simulink model "punto4y5"  (R2024a)
settings: Solver=VariableStepAuto  StartTime=0.0  StopTime=50  RelTol=1e-3
libraries: fuzblock x3, slpidlib x1
settings Model: Creator=USER  LastModifiedBy=USER

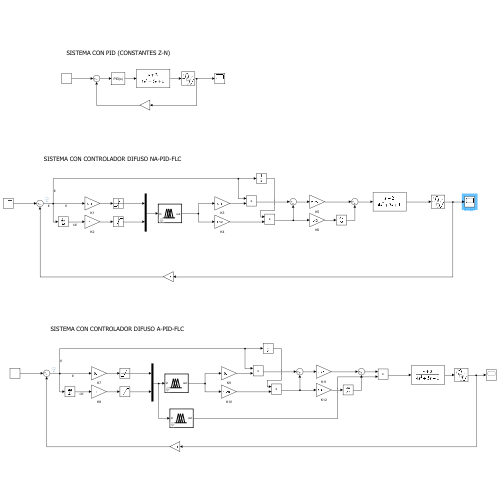
[thumbnail: Simulink's stored preview of the top-level diagram]
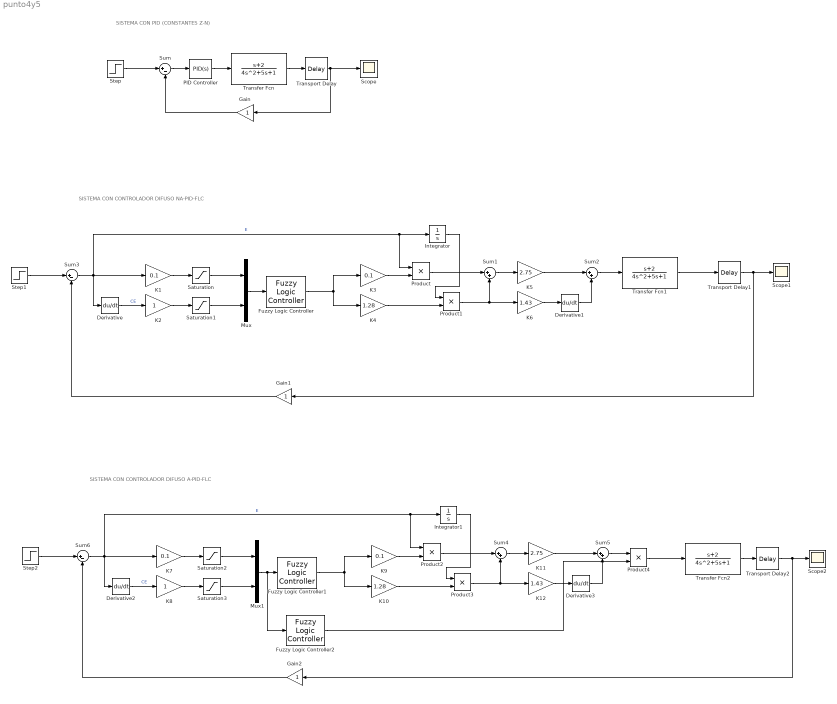
== system punto4y5 ==
  note: SISTEMA CON PID (CONSTANTES Z-N)
  note: SISTEMA CON CONTROLADOR DIFUSO NA-PID-FLC
  note: SISTEMA CON CONTROLADOR DIFUSO A-PID-FLC
  Derivative{,1..3} (4 alike) : Derivative
  Fuzzy Logic Controller : fuzblock/Fuzzy Logic  Controller  FIS='fuzzy_1.fis'  OutputSampleNumber=101  DataType=double  FuzzifiedInputs=off  RuleFiringStrengths=off  RuleOutputs=off  AggregatedOutputs=off  SimulateUsing=Interpreted execution  OutOfRangeInputValueMessage=warning  NoRuleFiredMessage=warning  EmptyOutputFuzzySetMessage=warning
  Fuzzy Logic Controller1 : fuzblock/Fuzzy Logic  Controller  FIS='fuzzy_1.fis'  OutputSampleNumber=101  DataType=double  FuzzifiedInputs=off  RuleFiringStrengths=off  RuleOutputs=off  AggregatedOutputs=off  SimulateUsing=Interpreted execution  OutOfRangeInputValueMessage=warning  NoRuleFiredMessage=warning  EmptyOutputFuzzySetMessage=warning
  Fuzzy Logic Controller2 : fuzblock/Fuzzy Logic  Controller  FIS='fuzzy_2.fis'  OutputSampleNumber=101  DataType=double  FuzzifiedInputs=off  RuleFiringStrengths=off  RuleOutputs=off  AggregatedOutputs=off  SimulateUsing=Interpreted execution  OutOfRangeInputValueMessage=warning  NoRuleFiredMessage=warning  EmptyOutputFuzzySetMessage=warning
  Gain : Gain
  Gain1 : Gain
  Gain2 : Gain
  Integrator : Integrator
  Integrator1 : Integrator
  K{1,3,7,9} (4 alike) : Gain  Gain=0.1
  K10 : Gain  Gain=1.28
  K11 : Gain  Gain=2.75
  K12 : Gain  Gain=1.43
  K2 : Gain
  K4 : Gain  Gain=1.28
  K5 : Gain  Gain=2.75
  K6 : Gain  Gain=1.43
  K8 : Gain
  Mux : Mux  Inputs=2
  Mux1 : Mux  Inputs=2
  PID Controller : slpidlib/PID Controller  Controller=PID  Form=Parallel  TimeDomain=Continuous-time  UseExternalTs=off  SampleTime=-1  IntegratorMethod=Forward Euler  FilterMethod=Forward Euler  ControllerParametersSource=internal  P=5.73  I=5  UseKiTs=off  D=1.43  UseExternalDerivativeSource=off  N=100  UseFilter=on  TunerSelectOption=Transfer Function Based (PID Tuner App)  InitialConditionSource=internal  InitialConditionForIntegrator=0  InitialConditionForFilter=0  DifferentiatorICPrevScaledInput=0  ExternalReset=none  TrackingMode=off  Kt=1  LimitOutput=off  SatLimitsSource=internal  UpperSaturationLimit=inf  LowerSaturationLimit=-inf  LinearizeAsGain=on  AntiWindupMode=none  Kb=1  LimitIntegrator=off  UpperIntegratorSaturationLimit=inf  LowerIntegratorSaturationLimit=-inf  POutMin=[]  POutMax=[]  IOutMin=[]  IOutMax=[]  DOutMin=[]  DOutMax=[]  NOutMin=[]  NOutMax=[]  SumOutMin=[]  SumOutMax=[]  SaturationOutMin=[]  SaturationOutMax=[]  PParamMin=[]  PParamMax=[]  IParamMin=[]  IParamMax=[]  DParamMin=[]  DParamMax=[]  NParamMin=[]  NParamMax=[]  KbParamMin=[]  KbParamMax=[]  KtParamMin=[]  KtParamMax=[]  KbOutMin=[]  KbOutMax=[]  KtOutMin=[]  KtOutMax=[]  IntegratorOutMin=[]  IntegratorOutMax=[]  FilterOutMin=[]  FilterOutMax=[]  SumI1OutMin=[]  SumI1OutMax=[]  SumI2OutMin=[]  SumI2OutMax=[]  SumI3OutMin=[]  SumI3OutMax=[]  SumI4OutMin=[]  SumI4OutMax=[]  SumDOutMin=[]  SumDOutMax=[]  DifferentiatorOutMin=[]  DifferentiatorOutMax=[]  FilterDiffOutCoefMin=[]  FilterDiffOutCoefMax=[]  ReciprocalOutMin=[]  ReciprocalOutMax=[]  SumDenOutMin=[]  SumDenOutMax=[]  SumNumOutMin=[]  SumNumOutMax=[]  DivideOutMin=[]  DivideOutMax=[]  UdiffTsProdOutMin=[]  UdiffTsProdOutMax=[]  NTsProdOutMin=[]  NTsProdOutMax=[]  UintegralTsProdOutMin=[]  UintegralTsProdOutMax=[]  UngainTsProdOutMin=[]  UngainTsProdOutMax=[]  ClampingZeroOutDataTypeStr=Inherit: Inherit via back propagation  ClampingZeroOutMin=[]  ClampingZeroOutMax=[]  FilterDenConstantOutDataTypeStr=Inherit: Inherit via back propagation  FilterDenConstantOutMin=[]  FilterDenConstantOutMax=[]  PCopyOutDataTypeStr=Inherit: Inherit via back propagation  PCopyOutMin=[]  PCopyOutMax=[]  NCopyOutDataTypeStr=Inherit: Inherit via back propagation  NCopyOutMin=[]  NCopyOutMax=[]  IntegratorContinuousStateAttributes=''  IntegratorStateMustResolveToSignalObject=off  IntegratorRTWStateStorageClass=Auto  FilterContinuousStateAttributes=''  FilterStateMustResolveToSignalObject=off  FilterRTWStateStorageClass=Auto  ParallelPVariant=InternalParameters  IdealPVariant=Disabled  IVariant=InternalParameters  DVariant=InternalParameters  IntegratorVariant=Continuous  SatVariant=Disabled  AWVariant=Passthrough  PCopyVariant=Disabled  TRVariant=Disabled  FdbkBlocksVariant=Forward  IdealPFdbkVariant=Disabled  SatFdbkVariant=Disabled  DerivativeFilterVariant=ContFilter  NVariant=InternalParameters  NCopyVariant=Disabled  FilterICVariant=InternalICsFilter  IntegratorICVariant=InternalICs  ExternalResetVariant=Disabled  TRSumVariant=Passthrough  SumFdbkVariant=Disabled  SumVariant=Sum_PID  TsampFilterVariant=InternalTs  TsampNgainVariant=Passthrough  TsampIntegralVariant=Disabled_SignalSpec  ExternalSaturationOutDataTypeStr=Inherit: Same as second input  DerivativeSourceVariant=ErrorSignal
  Product{,1..4} (5 alike) : Product
  Saturation{,1..3} (4 alike) : Saturate  UpperLimit=1  LowerLimit=-1
  Scope : Scope
  Scope1 : Scope
  Scope2 : Scope
  Step : Step  SampleTime=0
  Step1 : Step  SampleTime=0
  Step2 : Step  SampleTime=0
  Sum : Sum  Inputs=|+-
  Sum{1..2,4..5} (4 alike) : Sum  Inputs=|++
  Sum3 : Sum  Inputs=|+-
  Sum6 : Sum  Inputs=|+-
  Transfer Fcn : TransferFcn  Numerator=[1 2]  Denominator=[4 5 1]
  Transfer Fcn1 : TransferFcn  Numerator=[1 2]  Denominator=[4 5 1]
  Transfer Fcn2 : TransferFcn  Numerator=[1 2]  Denominator=[4 5 1]
  Transport Delay : TransportDelay  DelayTime=0.5
  Transport Delay1 : TransportDelay  DelayTime=0.5
  Transport Delay2 : TransportDelay  DelayTime=0.5
  wires:
  Sum/1 -> PID Controller/1
  Transfer Fcn/1 -> Transport Delay/1
  PID Controller/1 -> Transfer Fcn/1
  Transport Delay/1 -> Gain/1, Scope/1
  Step/1 -> Sum/1
  Gain/1 -> Sum/2
  K1/1 -> Saturation/1
  Derivative/1 -> K2/1  "CE"
  K2/1 -> Saturation1/1
  Saturation1/1 -> Mux/2
  Saturation/1 -> Mux/1
  Fuzzy Logic Controller/1 -> K4/1, K3/1
  K3/1 -> Product/2
  Sum3/1 -> Derivative/1, K1/1, Integrator/1, Product/1  "E"
  K4/1 -> Product1/2
  Integrator/1 -> Product1/1
  Product/1 -> Sum1/1
  Product1/1 -> K6/1, Sum1/2
  Sum1/1 -> K5/1
  K6/1 -> Derivative1/1
  K5/1 -> Sum2/1
  Derivative1/1 -> Sum2/2
  Step1/1 -> Sum3/1
  Sum2/1 -> Transfer Fcn1/1
  Transfer Fcn1/1 -> Transport Delay1/1
  Transport Delay1/1 -> Scope1/1, Gain1/1
  Gain1/1 -> Sum3/2
  Mux/1 -> Fuzzy Logic Controller/1
  Fuzzy Logic Controller1/1 -> K10/1, K9/1
  Mux1/1 -> Fuzzy Logic Controller2/1, Fuzzy Logic Controller1/1
  Sum6/1 -> Derivative2/1, K7/1, Integrator1/1, Product2/1  "E"
  Step2/1 -> Sum6/1
  Derivative3/1 -> Sum5/2
  Gain2/1 -> Sum6/2
  Transfer Fcn2/1 -> Transport Delay2/1
  Transport Delay2/1 -> Scope2/1, Gain2/1
  K12/1 -> Derivative3/1
  K9/1 -> Product2/2
  Integrator1/1 -> Product3/1
  K10/1 -> Product3/2
  Derivative2/1 -> K8/1  "CE"
  Product3/1 -> K12/1, Sum4/2
  Sum4/1 -> K11/1
  K8/1 -> Saturation3/1
  Saturation2/1 -> Mux1/1
  Saturation3/1 -> Mux1/2
  Product2/1 -> Sum4/1
  K11/1 -> Sum5/1
  K7/1 -> Saturation2/1
  Sum5/1 -> Product4/1
  Fuzzy Logic Controller2/1 -> Product4/2
  Product4/1 -> Transfer Fcn2/1
